simulink model "FitzHugh_Nagumo"  (R2019a)
settings: Solver=VariableStepAuto  StartTime=0.0  StopTime=1000  RelTol=1e-9
undefined symbols (not defined in the file or in its folder): sigbuilder_block
settings Model: Creator=Pranav Maddula  LastModifiedBy=Pranav Maddula

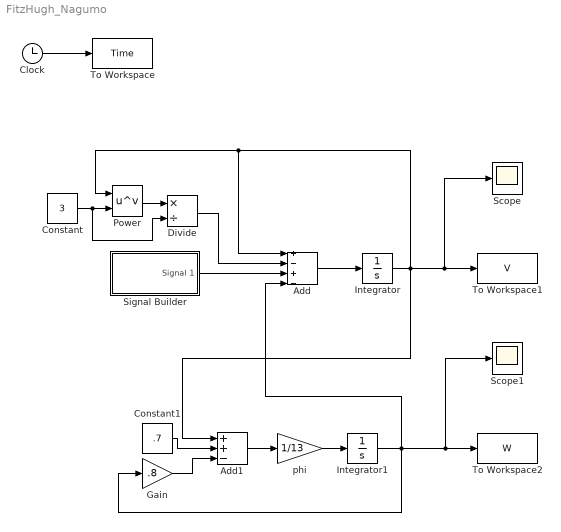
== system FitzHugh_Nagumo ==
  Add : Sum  Inputs=+-+-
  Add1 : Sum  Inputs=++-
  Clock : Clock
  Constant : Constant  Value=3
  Constant1 : Constant  Value=.7
  Divide : Product  Inputs=*/
  Gain : Gain  Gain=.8
  Integrator : Integrator
  Integrator1 : Integrator
  Power : Math  Operator=pow  SaturateOnIntegerOverflow=on
  Scope : Scope
  Scope1 : Scope
  Signal Builder : Subsystem  Tag=STV Subsys  LoadFcn=sigbuilder_block('load');  StartFcn=sigbuilder_block('start');  StopFcn=sigbuilder_block('stop');  ClipboardFcn=sigbuilder_block('clipboard');  mask(Sigbuilder block){tuvar=[0:10]}
      mask help: Simulink:masks:SigbuilderBlock_MD
      mask init:
      | if ~strcmp(get_param(bdroot(gcbh),'SimulationStatus'),'stopped') tuvar = sigbuilder_block('maskInit'); end
      settings: CopyFcn=sigbuilder_block('copy');  DeleteFcn=sigbuilder_block('delete');  ModelCloseFcn=sigbuilder_block('modelClose');  PreSaveFcn=sigbuilder_block('preSave');  PauseFcn=sigbuilder_block('pause');  ContinueFcn=sigbuilder_block('continue');  NameChangeFcn=sigbuilder_block('namechange');  OpenFcn=sigbuilder_block('open',[437.6 199.2 550.4 400 ]);  CloseFcn=sigbuilder_block('close');
      mask Display: plot(0, 0, 100, 100,[2, 2, 32, 32, 2], [68, 8, 8, 68, 68],[32, 2], [38, 38], [32, 19, 2],[53, 60, 44], [32, 17, 17, 2],[16, 16, 31, 31]);txt = getActiveGroup(gcbh);text(2, 100, txt,'verticalAlignment', 'top');
  To Workspace : ToWorkspace  VariableName=Time  SampleTime=-1
  To Workspace1 : ToWorkspace  VariableName=V  SampleTime=-1
  To Workspace2 : ToWorkspace  VariableName=W  SampleTime=-1
  phi : Gain  Gain=1/13
  wires:
  Integrator/1 -> Add/1, Power/1, Scope/1, To Workspace1/1, Add1/1
  Constant/1 -> Divide/2, Power/2
  Add/1 -> Integrator/1
  Power/1 -> Divide/1
  Divide/1 -> Add/2
  Add1/1 -> phi/1
  Constant1/1 -> Add1/2
  Gain/1 -> Add1/3
  phi/1 -> Integrator1/1
  Integrator1/1 -> Scope1/1, To Workspace2/1, Gain/1, Add/4
  Clock/1 -> To Workspace/1
  Signal Builder/1(Signal 1) -> Add/3

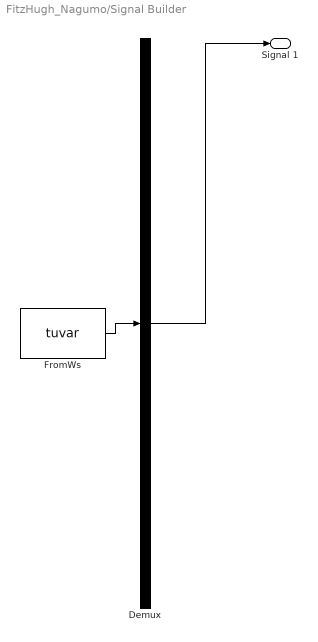
== system FitzHugh_Nagumo/Signal Builder ==
  Demux : Demux  Tag=STV Demux  Outputs=1
  FromWs : FromWorkspace  Tag=STV FromWs  VariableName=tuvar  SampleTime=0
      SigBuilderData=|
      | common.afterFinalStr = 'Extrapolate'
      | common.sampleTime = 0
      | dataSet.timeRange = [0 1000]
      | dataSet.name = 'Group 1'
      | sbobj.Groups.Name = 'Group 1'
      | sbobj.Groups.Signals.Name = 'Signal 1'
      | sbobj.Groups.Signals.XData = [0 10 1000]
      | sbobj.Groups.Signals.YData = [0 1 1]
      | sbobj.Groups.TimeRange = [0 1000]
  Signal 1 : Outport  Tag=STV Outport
  wires:
  Demux/1 -> Signal 1/1
  FromWs/1 -> Demux/1
